simulink model "mod3tb_ciff_2bit"  (Simulink 8.1)
settings: Solver=FixedStepDiscrete  StartTime=0.0  StopTime=10e-3  RelTol=1e-3
undefined symbols (not defined in the file): a, b, c, g, modctrl
libraries: dspsigops x3
settings Model: Creator=amyles  LastModifiedBy=amyles
settings DataIOCC: MaxDataPoints=50000
settings OptimizationCC: InlineParams=on
settings DebuggingCC: UnderspecifiedInitializationDetection=Simplified  InvalidFcnCallConnMsg=none  StrictBusMsg=ErrorOnBusTreatedAsVector
settings ModelReferenceCC: ModelReferenceNumInstancesAllowed=Single

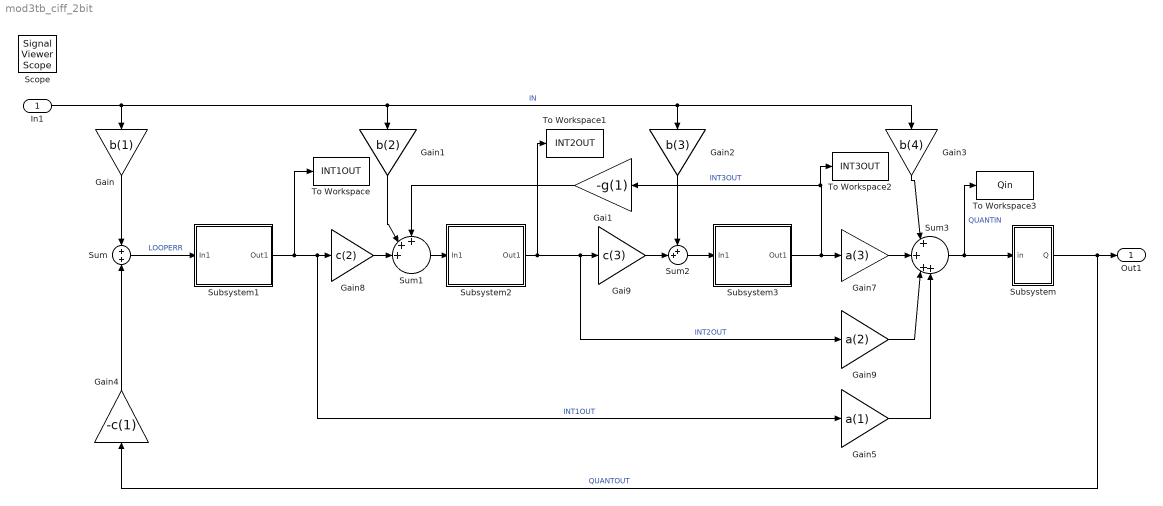
== system mod3tb_ciff_2bit ==
  In1 : Inport
  Gai1 : Gain  Gain=-g(1)
  Gai9 : Gain  Gain=c(3)
  Gain : Gain  Gain=b(1)
  Gain1 : Gain  Gain=b(2)
  Gain2 : Gain  Gain=b(3)
  Gain3 : Gain  Gain=b(4)
  Gain4 : Gain  Gain=-c(1)
  Gain5 : Gain  Gain=a(1)
  Gain7 : Gain  Gain=a(3)
  Gain8 : Gain  Gain=c(2)
  Gain9 : Gain  Gain=a(2)
  Subsystem : Subsystem
      settings: AttributesFormatString=2-bit quantiser
  Subsystem1 : Subsystem
      settings: AttributesFormatString=Leaky delaying integrator
  Subsystem2 : Subsystem
      settings: AttributesFormatString=Leaky delaying integrator
  Subsystem3 : Subsystem
      settings: AttributesFormatString=Leaky delaying integrator
  Sum : Sum
  Sum1 : Sum  Inputs=+++||
  Sum2 : Sum  Inputs=++|
  Sum3 : Sum  Inputs=|+|+|++
  To Workspace : ToWorkspace  VariableName=INT1OUT  SampleTime=-1
  To Workspace1 : ToWorkspace  VariableName=INT2OUT  SampleTime=-1
  To Workspace2 : ToWorkspace  VariableName=INT3OUT  SampleTime=-1
  To Workspace3 : ToWorkspace  VariableName=Qin  SampleTime=-1
  Out1 : Outport
  Scope : SignalViewerScope  IOType=viewer  NumInputPorts=6  ZoomMode=xonly  RefreshTime=0.035000
      settings: YMin=-5~-5~-5~-5~-5~-5  YMax=5~5~5~5~5~5
  wires:
  In1/1 -> Gain3/1, Gain2/1, Gain1/1, Gain/1  "IN"
  Subsystem1/1(Out1) -> To Workspace/1, Gain5/1, Gain8/1  "INT1OUT"
  Gain8/1 -> Sum1/3
  Subsystem2/1(Out1) -> To Workspace1/1, Gain9/1, Gai9/1  "INT2OUT"
  Gai9/1 -> Sum2/2
  Subsystem3/1(Out1) -> Gain7/1, To Workspace2/1, Gai1/1  "INT3OUT"
  Gain4/1 -> Sum/2
  Gain/1 -> Sum/1
  Gain1/1 -> Sum1/2
  Gai1/1 -> Sum1/1
  Gain2/1 -> Sum2/1
  Subsystem/1(Q) -> Out1/1, Gain4/1  "QUANTOUT"
  Sum/1 -> Subsystem1/1(In1)  "LOOPERR"
  Sum2/1 -> Subsystem3/1(In1)
  Sum1/1 -> Subsystem2/1(In1)
  Gain3/1 -> Sum3/1
  Gain7/1 -> Sum3/2
  Gain9/1 -> Sum3/3
  Gain5/1 -> Sum3/4
  Sum3/1 -> To Workspace3/1, Subsystem/1(in)  "QUANTIN"

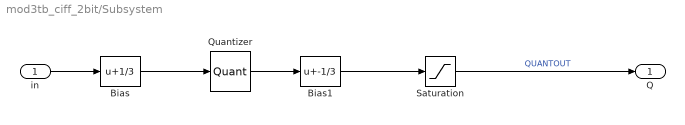
== system mod3tb_ciff_2bit/Subsystem ==
  in : Inport
  Bias : Bias  Bias=1/3
      settings: AttributesFormatString=Need offset to give\nMID-RISE quantiser
  Bias1 : Bias  Bias=-1/3
  Quantizer : Quantizer  QuantizationInterval=2/3  LinearizeAsGain=off
  Saturation : Saturate  UpperLimit=1  LowerLimit=-1
  Q : Outport
  wires:
  Bias/1 -> Quantizer/1
  Saturation/1 -> Q/1  "QUANTOUT"
  Quantizer/1 -> Bias1/1
  Bias1/1 -> Saturation/1
  in/1 -> Bias/1

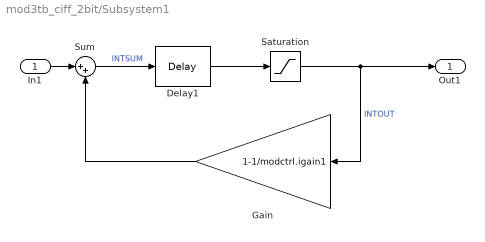
== system mod3tb_ciff_2bit/Subsystem1 ==
  In1 : Inport
  Delay1 : dspsigops/Delay  InputProcessing=Inherited (this choice will be removed - see release notes)  dly_unit=Samples  delay=1  ic_detail=off  dif_ic_for_ch=off  dif_ic_for_dly=off  ic=0  reset_popup=None
  Gain : Gain  Gain=1-1/modctrl.igain1
      settings: AttributesFormatString=Integrator leakage
  Saturation : Saturate  UpperLimit=modctrl.isat1  LowerLimit=-(modctrl.isat1)
  Sum : Sum  Inputs=|++
      settings: AttributesFormatString=Integrator summer
  Out1 : Outport
  wires:
  Sum/1 -> Delay1/1  "INTSUM"
  Gain/1 -> Sum/2
  Saturation/1 -> Gain/1, Out1/1  "INTOUT"
  In1/1 -> Sum/1
  Delay1/1 -> Saturation/1

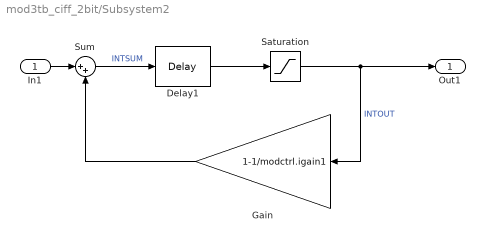
== system mod3tb_ciff_2bit/Subsystem2 ==
  In1 : Inport
  Delay1 : dspsigops/Delay  InputProcessing=Inherited (this choice will be removed - see release notes)  dly_unit=Samples  delay=1  ic_detail=off  dif_ic_for_ch=off  dif_ic_for_dly=off  ic=0  reset_popup=None
  Gain : Gain  Gain=1-1/modctrl.igain1
      settings: AttributesFormatString=Integrator leakage
  Saturation : Saturate  UpperLimit=modctrl.isat1  LowerLimit=-(modctrl.isat1)
  Sum : Sum  Inputs=|++
      settings: AttributesFormatString=Integrator summer
  Out1 : Outport
  wires:
  Sum/1 -> Delay1/1  "INTSUM"
  Gain/1 -> Sum/2
  Saturation/1 -> Gain/1, Out1/1  "INTOUT"
  In1/1 -> Sum/1
  Delay1/1 -> Saturation/1

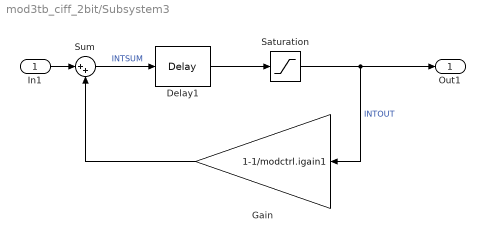
== system mod3tb_ciff_2bit/Subsystem3 ==
  In1 : Inport
  Delay1 : dspsigops/Delay  InputProcessing=Inherited (this choice will be removed - see release notes)  dly_unit=Samples  delay=1  ic_detail=off  dif_ic_for_ch=off  dif_ic_for_dly=off  ic=0  reset_popup=None
  Gain : Gain  Gain=1-1/modctrl.igain1
      settings: AttributesFormatString=Integrator leakage
  Saturation : Saturate  UpperLimit=modctrl.isat1  LowerLimit=-(modctrl.isat1)
  Sum : Sum  Inputs=|++
      settings: AttributesFormatString=Integrator summer
  Out1 : Outport
  wires:
  Sum/1 -> Delay1/1  "INTSUM"
  Gain/1 -> Sum/2
  Saturation/1 -> Gain/1, Out1/1  "INTOUT"
  In1/1 -> Sum/1
  Delay1/1 -> Saturation/1
